simulink library "TorqueCommand"  (R2024a)
settings: Solver=VariableStepAuto  StartTime=0.0  StopTime=10.0  RelTol=1e-3
undefined symbols (not defined in the file or in its folder): raptor_xcp_function
libraries: Raptor_lib x46, simulink x3, Utilities x2
settings Model: Creator=serga  LastModifiedBy=hyuga

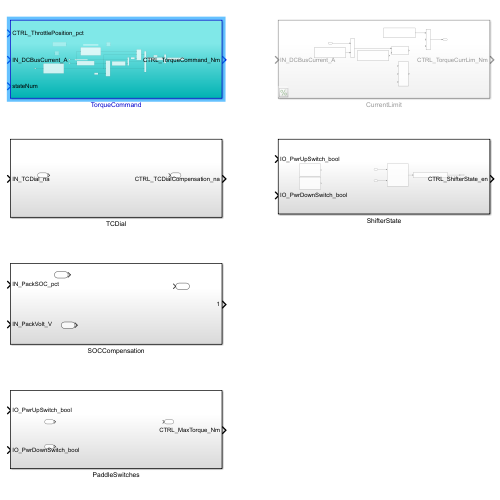
[thumbnail: Simulink's stored preview of the top-level diagram]
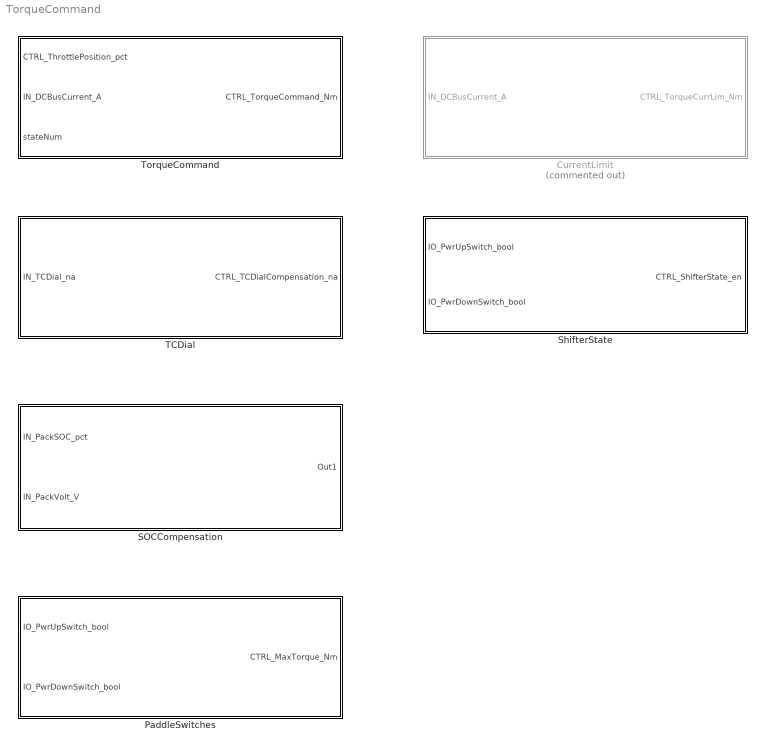
== system TorqueCommand ==
  CurrentLimit : Subsystem  Commented=on
  PaddleSwitches : Subsystem
  SOCCompensation : Subsystem
  ShifterState : Subsystem
  TCDial : Subsystem
  TorqueCommand : Subsystem

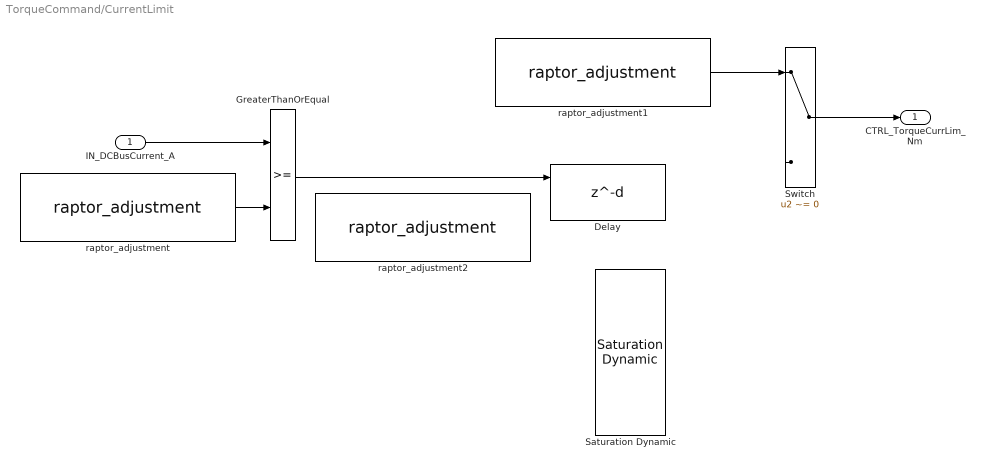
== system TorqueCommand/CurrentLimit ==
  IN_DCBusCurrent_A : Inport
  Delay : Delay  DelayLengthSource=Input port
      settings: InputPortMap=u0,p1
  GreaterThanOrEqual : RelationalOperator  OutDataTypeStr=boolean  RndMeth=Simplest  InputSameDT=off
  Saturation Dynamic : simulink/Discontinuities/Saturation Dynamic  OutMin=[]  OutMax=[]  OutDataTypeStr=Inherit: Same as second input  OutDataType=fixdt(1, 16)  OutScaling=2^-10  DoSatur=off
  Switch : Switch  Criteria=u2 ~= 0  SaturateOnIntegerOverflow=off  InputSameDT=off
  raptor_adjustment : Raptor_lib/Data Storage/raptor_adjustment  paramName='CTRL_DCBusOverCurrThresh_A'  nameSource=Parameter  initValue=125  dataType=uint8  storage=Calibration  calDispType=Number  calEnum={'False', 'True'}  calGain=1.0  calOffset=0.0  calMax=inf  calMin=-inf  calFormat='-1'  calUnit=''  calHelp=''  calAccess=1  calFunction=raptor_xcp_function(gcb)  calDispHeaders=off  calColHeaders={'Col1' 'Col2' 'Col3'}  calRowHeaders={'Row1' 'Row2' 'Row3'}
      settings: SourceProductName=Raptor
  raptor_adjustment1 : Raptor_lib/Data Storage/raptor_adjustment  paramName='CTRL_TorqueCurrLim_Nm'  nameSource=Parameter  initValue=100  dataType=double  storage=Calibration  calDispType=Number  calEnum={'False', 'True'}  calGain=1.0  calOffset=0.0  calMax=inf  calMin=-inf  calFormat='-1'  calUnit=''  calHelp=''  calAccess=1  calFunction=raptor_xcp_function(gcb)  calDispHeaders=off  calColHeaders={'Col1' 'Col2' 'Col3'}  calRowHeaders={'Row1' 'Row2' 'Row3'}
      settings: SourceProductName=Raptor
  raptor_adjustment2 : Raptor_lib/Data Storage/raptor_adjustment  paramName='CTRL_TorqueCurrLim_Nm'  nameSource=Parameter  initValue=100  dataType=double  storage=Calibration  calDispType=Number  calEnum={'False', 'True'}  calGain=1.0  calOffset=0.0  calMax=inf  calMin=-inf  calFormat='-1'  calUnit=''  calHelp=''  calAccess=1  calFunction=raptor_xcp_function(gcb)  calDispHeaders=off  calColHeaders={'Col1' 'Col2' 'Col3'}  calRowHeaders={'Row1' 'Row2' 'Row3'}
      settings: SourceProductName=Raptor
  CTRL_TorqueCurrLim_Nm : Outport
  wires:
  IN_DCBusCurrent_A/1 -> GreaterThanOrEqual/1
  raptor_adjustment/1 -> GreaterThanOrEqual/2
  GreaterThanOrEqual/1 -> Delay/1
  Switch/1 -> CTRL_TorqueCurrLim_Nm/1
  raptor_adjustment1/1 -> Switch/1

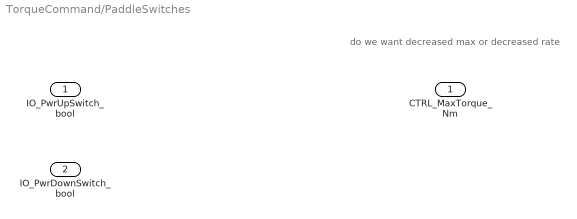
== system TorqueCommand/PaddleSwitches ==
  note: do we want decreased max or decreased rate
  IO_PwrUpSwitch_bool : Inport
  IO_PwrDownSwitch_bool : Inport  Port=2
  CTRL_MaxTorque_Nm : Outport

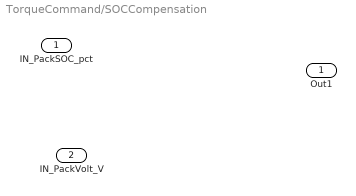
== system TorqueCommand/SOCCompensation ==
  IN_PackSOC_pct : Inport
  IN_PackVolt_V : Inport  Port=2
  Out1 : Outport

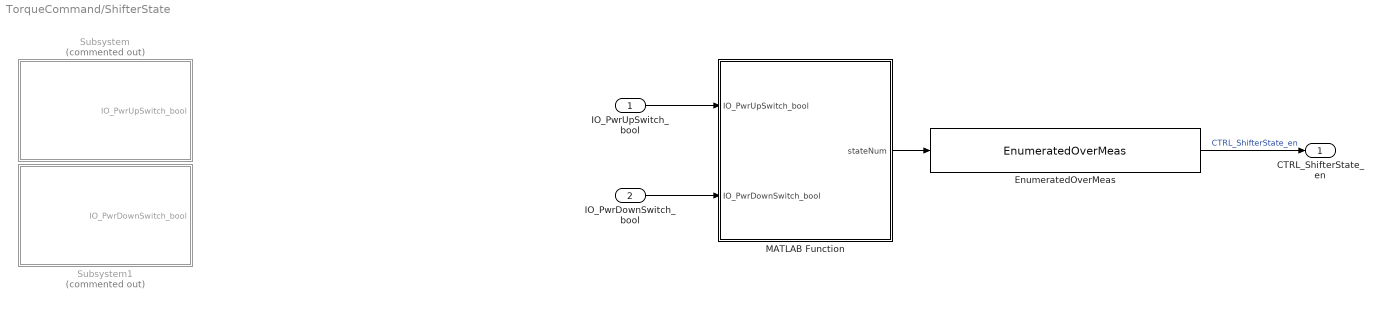
== system TorqueCommand/ShifterState ==
  IO_PwrUpSwitch_bool : Inport
  IO_PwrDownSwitch_bool : Inport  Port=2
  EnumeratedOverMeas : Utilities/EnumeratedOverMeas  sigName='CTRL_ShifterState_en'  enumName='TorqueState'
  MATLAB Function : MATLAB Function  TreatAsAtomicUnit=on
  Subsystem : Subsystem  Commented=on
  Subsystem1 : Subsystem  Commented=on
  CTRL_ShifterState_en : Outport
  wires:
  EnumeratedOverMeas/1 -> CTRL_ShifterState_en/1  "CTRL_ShifterState_en"
  MATLAB Function/1(stateNum) -> EnumeratedOverMeas/1
  IO_PwrDownSwitch_bool/1 -> MATLAB Function/2(IO_PwrDownSwitch_bool)
  IO_PwrUpSwitch_bool/1 -> MATLAB Function/1(IO_PwrUpSwitch_bool)

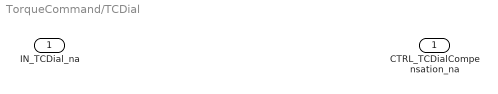
== system TorqueCommand/TCDial ==
  IN_TCDial_na : Inport
  CTRL_TCDialCompensation_na : Outport

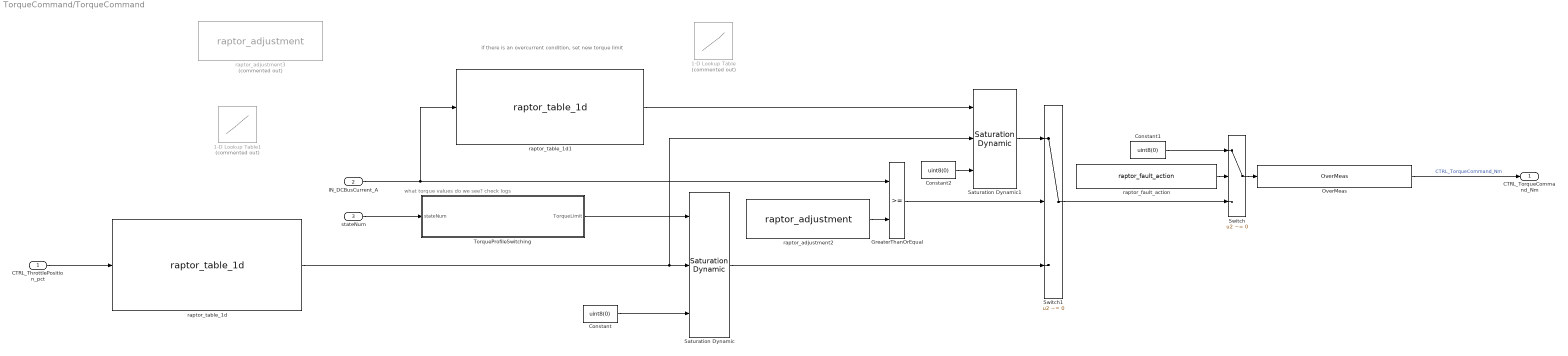
== system TorqueCommand/TorqueCommand ==
  note: if there is an overcurrent condition, set new torque limit
  note: what torque values do we see? check logs
  CTRL_ThrottlePosition_pct : Inport
  IN_DCBusCurrent_A : Inport  Port=2
  stateNum : Inport  Port=3
  1-D Lookup Table : Lookup_n-D  Commented=on  NumberOfTableDimensions=1  BreakpointsForDimension1=[0;5;10;15;20;25;30;35;40;45;50;55;60;65;70;75;80;85;90;95;100;105;110;115;120;125;130;135;140;145;150;155;160;165;170;175;180;185;190;195;200;205;210;215;220;225;230;235;240;245;250;255;260;265;270;275;280;285;290;295;300]  Table=[200;200;200;200;200;200;200;200;200;200;200;200;200;200;200;200;200;200;200;200;200;200;200;200;200;200;200;200;200;200;200;200;200;200;200;200;200;200;200;200;200;200;200;200;200;200;200;200;200;200;200;195;190;185;180;175;170;165;160;155;150]  InternalRulePriority=Speed  RndMeth=Simplest
  1-D Lookup Table1 : Lookup_n-D  Commented=on  NumberOfTableDimensions=1  BreakpointsForDimension1=[0;5;10;15;20;25;30;35;40;45;50;55;60;65;70;75;80;85;90;95;100]  Table=[0;3;6;9;12;15;25;35;45;55;65;75;85;95;105;115;135;155;175;195;200]  InternalRulePriority=Speed  RndMeth=Simplest
  Constant : Constant  Value=uint8(0)
  Constant1 : Constant  Value=uint8(0)
  Constant2 : Constant  Value=uint8(0)
  GreaterThanOrEqual : RelationalOperator  OutDataTypeStr=boolean  RndMeth=Simplest  InputSameDT=off
  OverMeas : Utilities/OverMeas  sigName='CTRL_TorqueCommand_Nm'  minimum=0  maximum=240
  Saturation Dynamic : simulink/Discontinuities/Saturation Dynamic  OutMin=[]  OutMax=[]  OutDataTypeStr=Inherit: Same as second input  OutDataType=fixdt(1, 16)  OutScaling=2^-10  DoSatur=off
  Saturation Dynamic1 : simulink/Discontinuities/Saturation Dynamic  OutMin=[]  OutMax=[]  OutDataTypeStr=Inherit: Same as second input  OutDataType=fixdt(1, 16)  OutScaling=2^-10  DoSatur=off
  Switch : Switch  Criteria=u2 ~= 0  SaturateOnIntegerOverflow=off  InputSameDT=off
  Switch1 : Switch  Criteria=u2 ~= 0  SaturateOnIntegerOverflow=off  InputSameDT=off
  TorqueProfileSwitching : Subsystem
  raptor_adjustment2 : Raptor_lib/Data Storage/raptor_adjustment  paramName='CTRL_DCBusOverCurrThresh_A'  nameSource=Parameter  initValue=125  dataType=single  storage=Calibration  calDispType=Number  calEnum={'False', 'True'}  calGain=1.0  calOffset=0.0  calMax=240  calMin=-inf  calFormat='-1'  calUnit=''  calHelp=''  calAccess=1  calFunction=raptor_xcp_function(gcb)  calDispHeaders=off  calColHeaders={'Col1' 'Col2' 'Col3'}  calRowHeaders={'Row1' 'Row2' 'Row3'}
      settings: SourceProductName=Raptor
  raptor_adjustment3 : Raptor_lib/Data Storage/raptor_adjustment  Commented=on  paramName='CTRL_TorqueCurrLim_Nm'  nameSource=Parameter  initValue=100  dataType=single  storage=Calibration  calDispType=Number  calEnum={'False', 'True'}  calGain=1.0  calOffset=0.0  calMax=inf  calMin=-inf  calFormat='-1'  calUnit=''  calHelp=''  calAccess=1  calFunction=raptor_xcp_function(gcb)  calDispHeaders=off  calColHeaders={'Col1' 'Col2' 'Col3'}  calRowHeaders={'Row1' 'Row2' 'Row3'}
      settings: SourceProductName=Raptor
  raptor_fault_action : Raptor_lib/Faults/raptor_fault_action  actionName='TorqueCmdOverride'  calVisible=on  calAccess=1  calFunction='System | FaultManager | FaultAction'
      settings: SourceProductName=Raptor
  raptor_table_1d : Raptor_lib/Table Lookup/raptor_table_1d  dataName='CTRL_ThrottleToTorqueCmd_1D'  initValue=[0;3;6;9;12;15;25;35;45;55;65;75;85;95;105;115;135;155;175;195;200]  dataType=single  storage=Calibration  initValueX=[0;5;10;15;20;25;30;35;40;45;50;55;60;65;70;75;80;85;90;95;100]  dataTypeXY=single  storageXY=Calibration  calVisible=on  showTable=on  calGain=1.0  calOffset=0.0  calMax=Inf  calMin=-Inf  calFormat='-1'  calUnit='pct'  calHelp=''  showBreakpoint=on  dataNameX=[]  calGainX=1.0  calOffsetX=0.0  calMaxX=Inf  calMinX=-Inf  calFormatX='-1'  calUnitX='Nm'  calHelpX=''  calAccess=1  calFunction=raptor_xcp_function(gcb)  measureEnable=off  mName=['Data1D_Output']
      settings: SourceProductName=Raptor
  raptor_table_1d1 : Raptor_lib/Table Lookup/raptor_table_1d  dataName='CTRL_ThrottleToLimTorqueCmd_1D'  initValue=[200;200;200;200;200;200;200;200;200;200;200;200;200;200;200;200;200;200;200;200;200;200;200;200;200;200;200;200;200;200;200;200;200;200;200;200;200;200;200;200;200;200;200;200;200;200;200;200;200;200;200;190;180;170;160;150;140;130;110;90;70]  dataType=single  storage=Calibration  initValueX=[0;5;10;15;20;25;30;35;40;45;50;55;60;65;70;75;80;85;90;95;100;105;110;115;120;125;130;135;140;145;150;155;160;165;170;175;180;185;190;195;200;205;210;215;220;225;230;235;240;245;250;255;260;265;270;275;280;285;290;295;300]  dataTypeXY=single  storageXY=Calibration  calVisible=on  showTable=on  calGain=1.0  calOffset=0.0  calMax=Inf  calMin=-Inf  calFormat='-1'  calUnit='Nm'  calHelp=''  showBreakpoint=on  dataNameX=[]  calGainX=1.0  calOffsetX=0.0  calMaxX=Inf  calMinX=-Inf  calFormatX='-1'  calUnitX='A'  calHelpX=''  calAccess=1  calFunction=raptor_xcp_function(gcb)  measureEnable=off  mName=['Data1D_Output']
      settings: SourceProductName=Raptor
  CTRL_TorqueCommand_Nm : Outport
  wires:
  stateNum/1 -> TorqueProfileSwitching/1(stateNum)
  TorqueProfileSwitching/1(TorqueLimit) -> Saturation Dynamic/1
  CTRL_ThrottlePosition_pct/1 -> raptor_table_1d/1
  raptor_table_1d/1 -> Saturation Dynamic/2, Saturation Dynamic1/2
  Constant/1 -> Saturation Dynamic/3
  Saturation Dynamic/1 -> Switch1/3
  Constant1/1 -> Switch/1
  Switch/1 -> OverMeas/1
  OverMeas/1 -> CTRL_TorqueCommand_Nm/1  "CTRL_TorqueCommand_Nm"
  raptor_fault_action/1 -> Switch/2
  Switch1/1 -> Switch/3
  raptor_adjustment2/1 -> GreaterThanOrEqual/2
  IN_DCBusCurrent_A/1 -> GreaterThanOrEqual/1, raptor_table_1d1/1
  GreaterThanOrEqual/1 -> Switch1/2
  Saturation Dynamic1/1 -> Switch1/1
  Constant2/1 -> Saturation Dynamic1/3
  raptor_table_1d1/1 -> Saturation Dynamic1/1

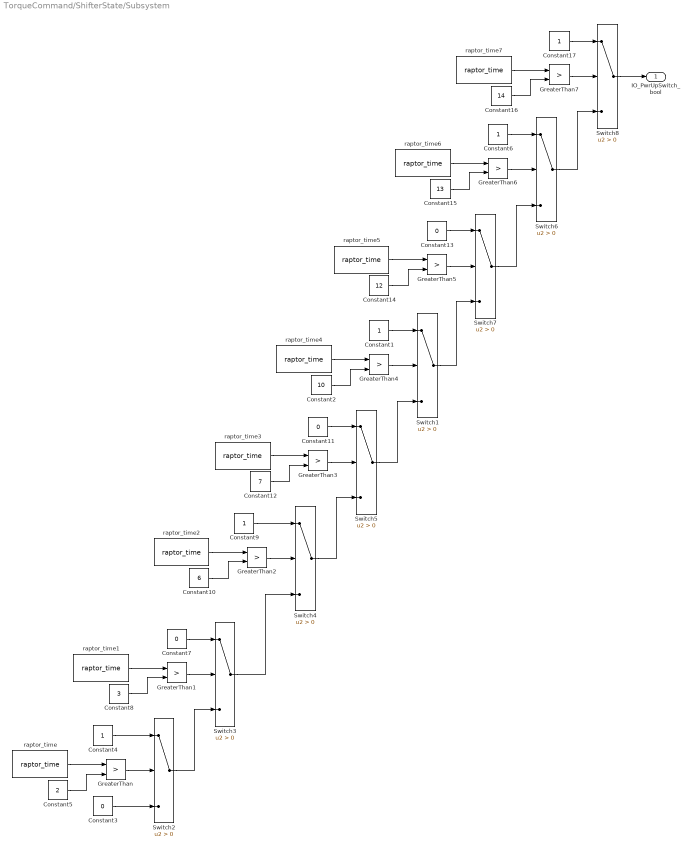
== system TorqueCommand/ShifterState/Subsystem ==
  Constant{1,4,6,9,17} (5 alike) : Constant
  Constant10 : Constant  Value=6
  Constant{3,7,11,13} (4 alike) : Constant  Value=0
  Constant12 : Constant  Value=7
  Constant14 : Constant  Value=12
  Constant15 : Constant  Value=13
  Constant16 : Constant  Value=14
  Constant2 : Constant  Value=10
  Constant5 : Constant  Value=2
  Constant8 : Constant  Value=3
  GreaterThan{,1..7} (8 alike) : RelationalOperator  Operator=>  OutDataTypeStr=boolean  RndMeth=Simplest  InputSameDT=off
  Switch{1..8} (8 alike) : Switch  Criteria=u2 > Threshold  SaturateOnIntegerOverflow=off  InputSameDT=off
  raptor_time{,1..7} (8 alike) : Raptor_lib/Triggers/raptor_time  unit=seconds
      settings: SourceProductName=Raptor
  IO_PwrUpSwitch_bool : Outport
  wires:
  Switch8/1 -> IO_PwrUpSwitch_bool/1
  GreaterThan7/1 -> Switch8/2
  Switch6/1 -> Switch8/3
  Constant16/1 -> GreaterThan7/2
  Constant17/1 -> Switch8/1
  raptor_time7/1 -> GreaterThan7/1
  Switch1/1 -> Switch7/3
  Constant14/1 -> GreaterThan5/2
  Constant15/1 -> GreaterThan6/2
  raptor_time5/1 -> GreaterThan5/1
  Constant6/1 -> Switch6/1
  GreaterThan5/1 -> Switch7/2
  GreaterThan6/1 -> Switch6/2
  raptor_time6/1 -> GreaterThan6/1
  Switch7/1 -> Switch6/3
  Constant13/1 -> Switch7/1
  Constant2/1 -> GreaterThan4/2
  Switch5/1 -> Switch1/3
  raptor_time4/1 -> GreaterThan4/1
  GreaterThan4/1 -> Switch1/2
  Constant1/1 -> Switch1/1
  Constant11/1 -> Switch5/1
  Constant8/1 -> GreaterThan1/2
  raptor_time1/1 -> GreaterThan1/1
  GreaterThan1/1 -> Switch3/2
  Switch4/1 -> Switch5/3
  GreaterThan3/1 -> Switch5/2
  raptor_time3/1 -> GreaterThan3/1
  raptor_time2/1 -> GreaterThan2/1
  Switch3/1 -> Switch4/3
  Constant10/1 -> GreaterThan2/2
  raptor_time/1 -> GreaterThan/1
  GreaterThan/1 -> Switch2/2
  Constant9/1 -> Switch4/1
  Constant5/1 -> GreaterThan/2
  Constant7/1 -> Switch3/1
  Constant3/1 -> Switch2/3
  Constant4/1 -> Switch2/1
  Switch2/1 -> Switch3/3
  Constant12/1 -> GreaterThan3/2
  GreaterThan2/1 -> Switch4/2

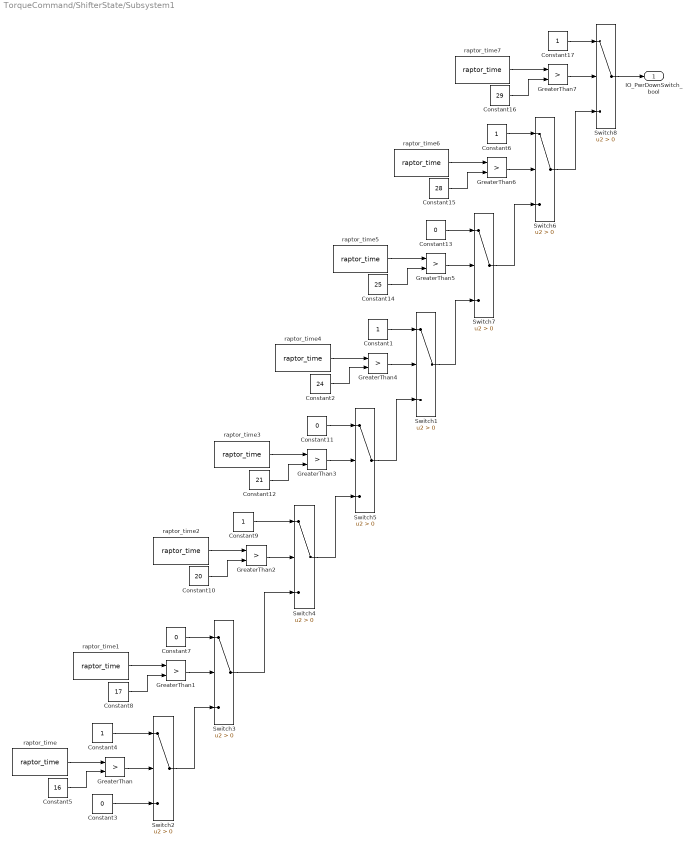
== system TorqueCommand/ShifterState/Subsystem1 ==
  Constant{1,4,6,9,17} (5 alike) : Constant
  Constant10 : Constant  Value=20
  Constant{3,7,11,13} (4 alike) : Constant  Value=0
  Constant12 : Constant  Value=21
  Constant14 : Constant  Value=25
  Constant15 : Constant  Value=28
  Constant16 : Constant  Value=29
  Constant2 : Constant  Value=24
  Constant5 : Constant  Value=16
  Constant8 : Constant  Value=17
  GreaterThan{,1..7} (8 alike) : RelationalOperator  Operator=>  OutDataTypeStr=boolean  RndMeth=Simplest  InputSameDT=off
  Switch{1..8} (8 alike) : Switch  Criteria=u2 > Threshold  SaturateOnIntegerOverflow=off  InputSameDT=off
  raptor_time{,1..7} (8 alike) : Raptor_lib/Triggers/raptor_time  unit=seconds
      settings: SourceProductName=Raptor
  IO_PwrDownSwitch_bool : Outport
  wires:
  Switch8/1 -> IO_PwrDownSwitch_bool/1
  GreaterThan7/1 -> Switch8/2
  Switch6/1 -> Switch8/3
  Constant16/1 -> GreaterThan7/2
  Constant17/1 -> Switch8/1
  raptor_time7/1 -> GreaterThan7/1
  Switch1/1 -> Switch7/3
  Constant14/1 -> GreaterThan5/2
  Constant15/1 -> GreaterThan6/2
  raptor_time5/1 -> GreaterThan5/1
  Constant6/1 -> Switch6/1
  GreaterThan5/1 -> Switch7/2
  GreaterThan6/1 -> Switch6/2
  raptor_time6/1 -> GreaterThan6/1
  Switch7/1 -> Switch6/3
  Constant13/1 -> Switch7/1
  Constant2/1 -> GreaterThan4/2
  Switch5/1 -> Switch1/3
  raptor_time4/1 -> GreaterThan4/1
  GreaterThan4/1 -> Switch1/2
  Constant1/1 -> Switch1/1
  Constant11/1 -> Switch5/1
  Constant8/1 -> GreaterThan1/2
  raptor_time1/1 -> GreaterThan1/1
  GreaterThan1/1 -> Switch3/2
  Switch4/1 -> Switch5/3
  GreaterThan3/1 -> Switch5/2
  raptor_time3/1 -> GreaterThan3/1
  raptor_time2/1 -> GreaterThan2/1
  Switch3/1 -> Switch4/3
  Constant10/1 -> GreaterThan2/2
  raptor_time/1 -> GreaterThan/1
  GreaterThan/1 -> Switch2/2
  Constant9/1 -> Switch4/1
  Constant5/1 -> GreaterThan/2
  Constant7/1 -> Switch3/1
  Constant3/1 -> Switch2/3
  Constant4/1 -> Switch2/1
  Switch2/1 -> Switch3/3
  Constant12/1 -> GreaterThan3/2
  GreaterThan2/1 -> Switch4/2

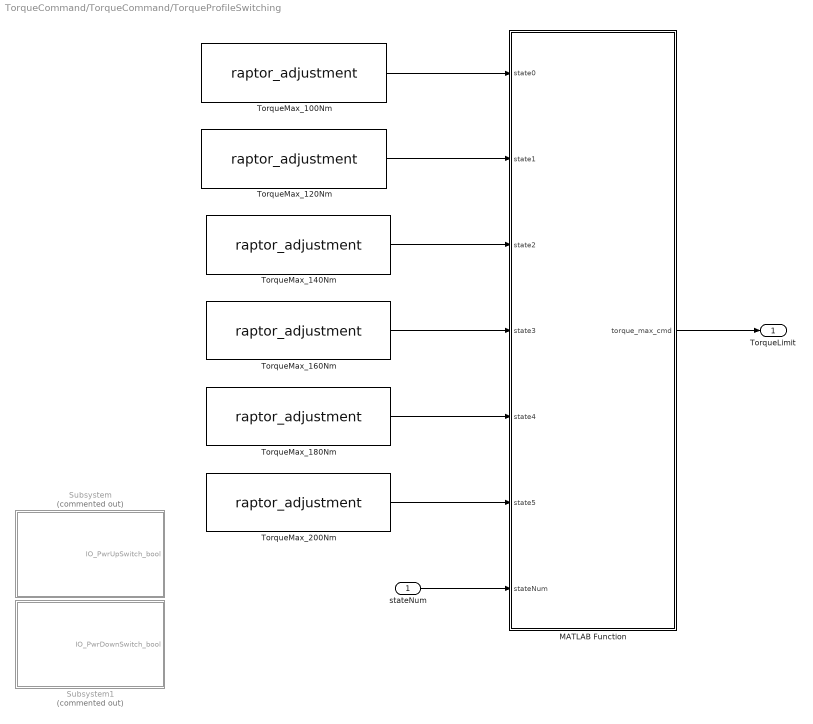
== system TorqueCommand/TorqueCommand/TorqueProfileSwitching ==
  stateNum : Inport
  MATLAB Function : MATLAB Function  TreatAsAtomicUnit=on
  Subsystem : Subsystem  Commented=on
  Subsystem1 : Subsystem  Commented=on
  TorqueMax_100Nm : Raptor_lib/Data Storage/raptor_adjustment  paramName='CTRL_TorqueCommandMax_100Nm'  nameSource=Parameter  initValue=100  dataType=single  storage=Calibration  calDispType=Number  calEnum={'False', 'True'}  calGain=1.0  calOffset=0.0  calMax=240  calMin=0  calFormat='-1'  calUnit=''  calHelp=''  calAccess=1  calFunction=raptor_xcp_function(gcb)  calDispHeaders=off  calColHeaders={'Col1' 'Col2' 'Col3'}  calRowHeaders={'Row1' 'Row2' 'Row3'}
      settings: SourceProductName=Raptor
  TorqueMax_120Nm : Raptor_lib/Data Storage/raptor_adjustment  paramName='CTRL_TorqueCommandMax_120Nm'  nameSource=Parameter  initValue=120  dataType=single  storage=Calibration  calDispType=Number  calEnum={'False', 'True'}  calGain=1.0  calOffset=0.0  calMax=240  calMin=0  calFormat='-1'  calUnit=''  calHelp=''  calAccess=1  calFunction=raptor_xcp_function(gcb)  calDispHeaders=off  calColHeaders={'Col1' 'Col2' 'Col3'}  calRowHeaders={'Row1' 'Row2' 'Row3'}
      settings: SourceProductName=Raptor
  TorqueMax_140Nm : Raptor_lib/Data Storage/raptor_adjustment  paramName='CTRL_TorqueCommandMax_140Nm'  nameSource=Parameter  initValue=140  dataType=single  storage=Calibration  calDispType=Number  calEnum={'False', 'True'}  calGain=1.0  calOffset=0.0  calMax=240  calMin=0  calFormat='-1'  calUnit=''  calHelp=''  calAccess=1  calFunction=raptor_xcp_function(gcb)  calDispHeaders=off  calColHeaders={'Col1' 'Col2' 'Col3'}  calRowHeaders={'Row1' 'Row2' 'Row3'}
      settings: SourceProductName=Raptor
  TorqueMax_160Nm : Raptor_lib/Data Storage/raptor_adjustment  paramName='CTRL_TorqueCommandMax_160Nm'  nameSource=Parameter  initValue=160  dataType=single  storage=Calibration  calDispType=Number  calEnum={'False', 'True'}  calGain=1.0  calOffset=0.0  calMax=240  calMin=0  calFormat='-1'  calUnit=''  calHelp=''  calAccess=1  calFunction=raptor_xcp_function(gcb)  calDispHeaders=off  calColHeaders={'Col1' 'Col2' 'Col3'}  calRowHeaders={'Row1' 'Row2' 'Row3'}
      settings: SourceProductName=Raptor
  TorqueMax_180Nm : Raptor_lib/Data Storage/raptor_adjustment  paramName='CTRL_TorqueCommandMax_180Nm'  nameSource=Parameter  initValue=180  dataType=single  storage=Calibration  calDispType=Number  calEnum={'False', 'True'}  calGain=1.0  calOffset=0.0  calMax=240  calMin=0  calFormat='-1'  calUnit=''  calHelp=''  calAccess=1  calFunction=raptor_xcp_function(gcb)  calDispHeaders=off  calColHeaders={'Col1' 'Col2' 'Col3'}  calRowHeaders={'Row1' 'Row2' 'Row3'}
      settings: SourceProductName=Raptor
  TorqueMax_200Nm : Raptor_lib/Data Storage/raptor_adjustment  paramName='CTRL_TorqueCommandMax_200Nm'  nameSource=Parameter  initValue=200  dataType=single  storage=Calibration  calDispType=Number  calEnum={'False', 'True'}  calGain=1.0  calOffset=0.0  calMax=240  calMin=0  calFormat='-1'  calUnit=''  calHelp=''  calAccess=1  calFunction=raptor_xcp_function(gcb)  calDispHeaders=off  calColHeaders={'Col1' 'Col2' 'Col3'}  calRowHeaders={'Row1' 'Row2' 'Row3'}
      settings: SourceProductName=Raptor
  TorqueLimit : Outport
  wires:
  stateNum/1 -> MATLAB Function/7(stateNum)
  MATLAB Function/1(torque_max_cmd) -> TorqueLimit/1
  TorqueMax_100Nm/1 -> MATLAB Function/1(state0)
  TorqueMax_120Nm/1 -> MATLAB Function/2(state1)
  TorqueMax_160Nm/1 -> MATLAB Function/4(state3)
  TorqueMax_140Nm/1 -> MATLAB Function/3(state2)
  TorqueMax_180Nm/1 -> MATLAB Function/5(state4)
  TorqueMax_200Nm/1 -> MATLAB Function/6(state5)

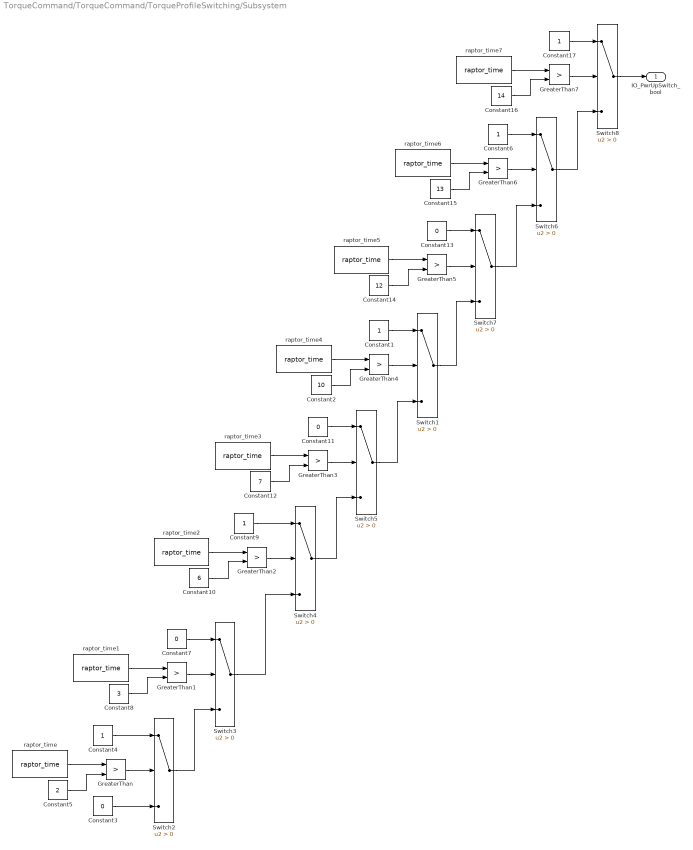
== system TorqueCommand/TorqueCommand/TorqueProfileSwitching/Subsystem ==
  Constant{1,4,6,9,17} (5 alike) : Constant
  Constant10 : Constant  Value=6
  Constant{3,7,11,13} (4 alike) : Constant  Value=0
  Constant12 : Constant  Value=7
  Constant14 : Constant  Value=12
  Constant15 : Constant  Value=13
  Constant16 : Constant  Value=14
  Constant2 : Constant  Value=10
  Constant5 : Constant  Value=2
  Constant8 : Constant  Value=3
  GreaterThan{,1..7} (8 alike) : RelationalOperator  Operator=>  OutDataTypeStr=boolean  RndMeth=Simplest  InputSameDT=off
  Switch{1..8} (8 alike) : Switch  Criteria=u2 > Threshold  SaturateOnIntegerOverflow=off  InputSameDT=off
  raptor_time{,1..7} (8 alike) : Raptor_lib/Triggers/raptor_time  unit=seconds
      settings: SourceProductName=Raptor
  IO_PwrUpSwitch_bool : Outport
  wires:
  Switch8/1 -> IO_PwrUpSwitch_bool/1
  GreaterThan7/1 -> Switch8/2
  Switch6/1 -> Switch8/3
  Constant16/1 -> GreaterThan7/2
  Constant17/1 -> Switch8/1
  raptor_time7/1 -> GreaterThan7/1
  Switch1/1 -> Switch7/3
  Constant14/1 -> GreaterThan5/2
  Constant15/1 -> GreaterThan6/2
  raptor_time5/1 -> GreaterThan5/1
  Constant6/1 -> Switch6/1
  GreaterThan5/1 -> Switch7/2
  GreaterThan6/1 -> Switch6/2
  raptor_time6/1 -> GreaterThan6/1
  Switch7/1 -> Switch6/3
  Constant13/1 -> Switch7/1
  Constant2/1 -> GreaterThan4/2
  Switch5/1 -> Switch1/3
  raptor_time4/1 -> GreaterThan4/1
  GreaterThan4/1 -> Switch1/2
  Constant1/1 -> Switch1/1
  Constant11/1 -> Switch5/1
  Constant8/1 -> GreaterThan1/2
  raptor_time1/1 -> GreaterThan1/1
  GreaterThan1/1 -> Switch3/2
  Switch4/1 -> Switch5/3
  GreaterThan3/1 -> Switch5/2
  raptor_time3/1 -> GreaterThan3/1
  raptor_time2/1 -> GreaterThan2/1
  Switch3/1 -> Switch4/3
  Constant10/1 -> GreaterThan2/2
  raptor_time/1 -> GreaterThan/1
  GreaterThan/1 -> Switch2/2
  Constant9/1 -> Switch4/1
  Constant5/1 -> GreaterThan/2
  Constant7/1 -> Switch3/1
  Constant3/1 -> Switch2/3
  Constant4/1 -> Switch2/1
  Switch2/1 -> Switch3/3
  Constant12/1 -> GreaterThan3/2
  GreaterThan2/1 -> Switch4/2

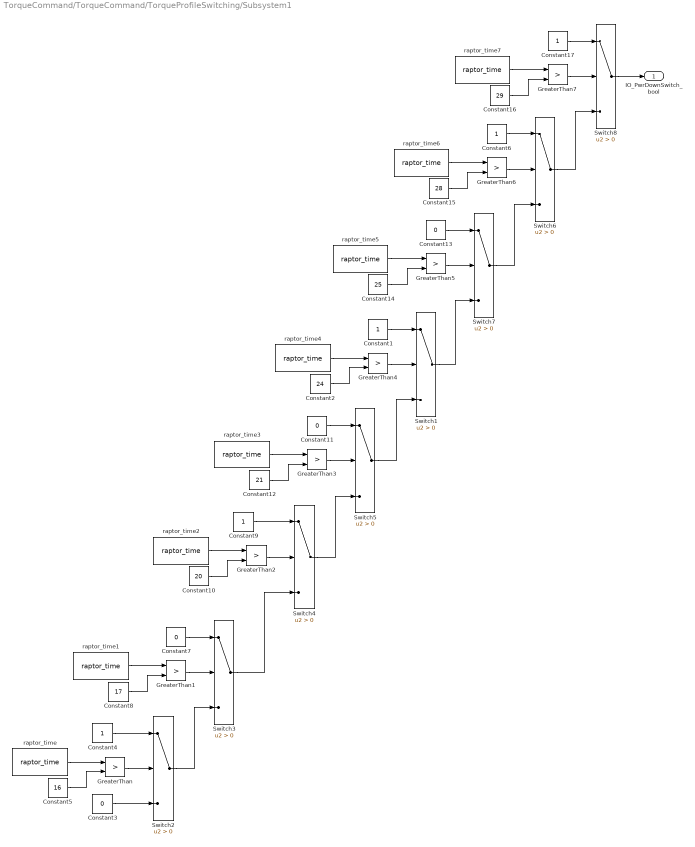
== system TorqueCommand/TorqueCommand/TorqueProfileSwitching/Subsystem1 ==
  Constant{1,4,6,9,17} (5 alike) : Constant
  Constant10 : Constant  Value=20
  Constant{3,7,11,13} (4 alike) : Constant  Value=0
  Constant12 : Constant  Value=21
  Constant14 : Constant  Value=25
  Constant15 : Constant  Value=28
  Constant16 : Constant  Value=29
  Constant2 : Constant  Value=24
  Constant5 : Constant  Value=16
  Constant8 : Constant  Value=17
  GreaterThan{,1..7} (8 alike) : RelationalOperator  Operator=>  OutDataTypeStr=boolean  RndMeth=Simplest  InputSameDT=off
  Switch{1..8} (8 alike) : Switch  Criteria=u2 > Threshold  SaturateOnIntegerOverflow=off  InputSameDT=off
  raptor_time{,1..7} (8 alike) : Raptor_lib/Triggers/raptor_time  unit=seconds
      settings: SourceProductName=Raptor
  IO_PwrDownSwitch_bool : Outport
  wires:
  Switch8/1 -> IO_PwrDownSwitch_bool/1
  GreaterThan7/1 -> Switch8/2
  Switch6/1 -> Switch8/3
  Constant16/1 -> GreaterThan7/2
  Constant17/1 -> Switch8/1
  raptor_time7/1 -> GreaterThan7/1
  Switch1/1 -> Switch7/3
  Constant14/1 -> GreaterThan5/2
  Constant15/1 -> GreaterThan6/2
  raptor_time5/1 -> GreaterThan5/1
  Constant6/1 -> Switch6/1
  GreaterThan5/1 -> Switch7/2
  GreaterThan6/1 -> Switch6/2
  raptor_time6/1 -> GreaterThan6/1
  Switch7/1 -> Switch6/3
  Constant13/1 -> Switch7/1
  Constant2/1 -> GreaterThan4/2
  Switch5/1 -> Switch1/3
  raptor_time4/1 -> GreaterThan4/1
  GreaterThan4/1 -> Switch1/2
  Constant1/1 -> Switch1/1
  Constant11/1 -> Switch5/1
  Constant8/1 -> GreaterThan1/2
  raptor_time1/1 -> GreaterThan1/1
  GreaterThan1/1 -> Switch3/2
  Switch4/1 -> Switch5/3
  GreaterThan3/1 -> Switch5/2
  raptor_time3/1 -> GreaterThan3/1
  raptor_time2/1 -> GreaterThan2/1
  Switch3/1 -> Switch4/3
  Constant10/1 -> GreaterThan2/2
  raptor_time/1 -> GreaterThan/1
  GreaterThan/1 -> Switch2/2
  Constant9/1 -> Switch4/1
  Constant5/1 -> GreaterThan/2
  Constant7/1 -> Switch3/1
  Constant3/1 -> Switch2/3
  Constant4/1 -> Switch2/1
  Switch2/1 -> Switch3/3
  Constant12/1 -> GreaterThan3/2
  GreaterThan2/1 -> Switch4/2

== matlab function TorqueCommand/ShifterState/MATLAB Function ==
  data: IO_PwrUpSwitch_bool input; IO_PwrDownSwitch_bool input; stateNum output
function stateNum  = fcn(IO_PwrUpSwitch_bool, IO_PwrDownSwitch_bool)

persistent state prevUp prevDown
if isempty(state)
    state = torqueState.state0;
end
if isempty(prevUp)
    prevUp = false;
    prevDown = false;
end
 
upButton = logical(IO_PwrUpSwitch_bool);
downButton = logical(IO_PwrDownSwitch_bool);
 
upEdge = (upButton && ~prevUp);
downEdge = (downButton && ~prevDown);
 
if upEdge
    newValue = min(uint8(state) + 1, 5);
    state = torqueState(newValue);
elseif downEdge
    newValue = max(uint8(state) - 1, 0);
    state = torqueState(newValue);
end
 
stateNum = uint8(state);
 
prevUp = upButton;
prevDown = downButton;

== matlab function TorqueCommand/TorqueProfileSwitching/MATLAB Function ==
  data: state0 input; torque_max_cmd output; state1 input; state2 input; state3 input; state4 input; state5 input; stateNum input
function torque_max_cmd = fcn(state0, state1, state2, state3, state4, state5, stateNum)
% Select torque limit based on numeric state (0–5)
 
switch uint8(stateNum)
    case 0
        torque_max_cmd = state0;
    case 1
        torque_max_cmd = state1;
    case 2
        torque_max_cmd = state2;
    case 3
        torque_max_cmd = state3;
    case 4
        torque_max_cmd = state4;
    case 5
        torque_max_cmd = state5;
    otherwise
        torque_max_cmd = state0;
end
